simulink model "PFC_MultiAxisKit_Sim"  (R2021b)
settings: Solver=VariableStepAuto  StartTime=0.0  StopTime=0.2  RelTol=1e-3
InitFcn:
  | run('PFC_MultiAxisKit_Param.m')
values from neighbouring files (symbols this model uses):
  f_PWM = 100000    [PFC_MultiAxisKit_Param.m]
  Ts_plant = 2e-7    (= 2e-07)    [PFC_MultiAxisKit_Param.m]
libraries: fl_lib x20, nesl_utility x7, tiiqmathlib x3, c28xdmclib x2, demo_controls x1, ee_lib x1, eePwmGenerator x1
CloseFcn:
  | clear('C_boost','C_filter','f_PWM','fin','L_boost','Ts','Vin_peak','PFC_Results','Ts_control','Ts_plant')
settings Model: Creator=The MathWorks, Inc.  LastModifiedBy=The MathWorks, Inc.
settings SolverCC: AlgebraicLoopSolver=TrustRegion
settings DataIOCC: SaveFormat=StructureWithTime  SaveTime=off  ReturnWorkspaceOutputs=off
settings DebuggingCC: ParameterPrecisionLossMsg=none  SymbolicDimsDataTypeCodeGenerationDiagnostic=none  SFMachineParentedDataDiag=warning

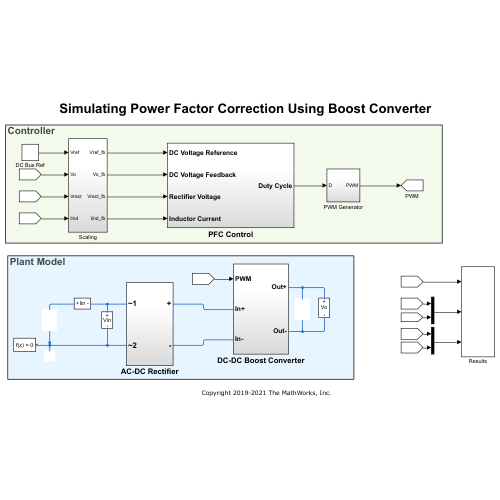
[thumbnail: Simulink's stored preview of the top-level diagram]
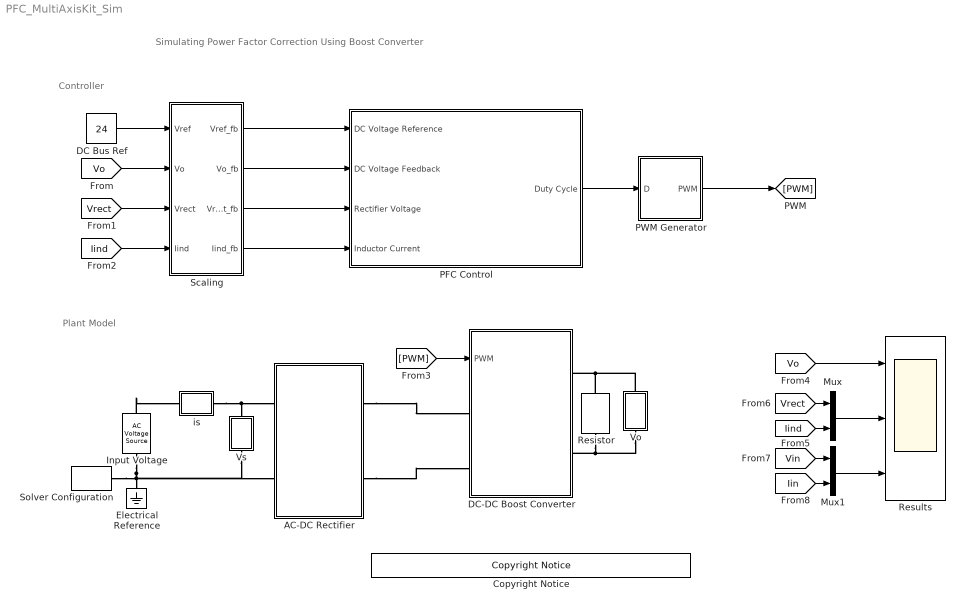
== system PFC_MultiAxisKit_Sim ==
  note: Controller
  note: Plant Model
  note: Simulating Power Factor Correction Using Boost Converter
  AC-DC Rectifier : Subsystem
  Copyright Notice : demo_controls/Copyright Notice  year=2019  prod=tic6000
      settings: SourceProductBaseCode=ME
  DC Bus Ref : Constant  Value=24  SampleTime=2e-5
  DC-DC Boost Converter : Subsystem
  Electrical Reference : fl_lib/Electrical/Electrical Elements/Electrical Reference
  Input Voltage : fl_lib/Electrical/Electrical Sources/AC Voltage Source  amp=Vin_peak V  shift=0 deg  frequency=fin Hz  omega=0 rad/s
  Mux : Mux  Inputs=2
  Mux1 : Mux  Inputs=2
  PFC Control : Subsystem
  PWM Generator : Subsystem
  Resistor : fl_lib/Electrical/Electrical Elements/Resistor  R=15.3 Ohm  i_specify=off  i_priority=None  i=0 A  i_nominal_specify=off  i_nominal_unit=A  i_nominal_value=1  v_specify=off  v_priority=None  v=0 V  v_nominal_specify=off  v_nominal_unit=V  v_nominal_value=1
  Results : Scope  NumInputPorts=3
  Scaling : Subsystem
  Solver Configuration : nesl_utility/Solver Configuration  PhysicalDomain=network_engine_domain  SubClassName=solver  LeftPortType=input  RightPortType=generic  Tones=[]  Harmonics=[]  SimulateNoise=off  Profile=off  UseLocalSampling=off  EnableSwitchedLinearOptims=on  FrequencyDomain=off  UseCCode=off  RelTol=0.001  AbsTol=1e-06  MinStep=1e-09  ToWorkspace=off  RevertToSquareIcSolve=off  NumHomotopyIterations=100  PhasorMode=off  PhasorModeNumHarmonics=1  DoDC=off  ResidualTolerance=1e-09  UseLocalSolver=on  LocalSolverChoice=NE_BACKWARD_EULER_ADVANCER  LocalSolverSampleTime=Ts_plant  DoFixedCost=on  MaxNonlinIter=4  MaxModeIter=2  ComputeImpulses=off  ImpulseIterations=2  LinearAlgebra=auto  EquationFormulation=NE_TIME_EF  DelaysMemoryBudget=1024  AutomaticFiltering=on  FilteringTimeConstant=0.001  PartitionStorageMethod=AS_NEEDED  PartitionMemoryBudget=1024  PartitionMethod=FAST
      settings: SourceProductBaseCode=PW,SS
  Vo : Subsystem
      mask Display:
      | disp('Vo')
      | port_label('Lconn',1,'+')
      | port_label('Rconn',1,'-')
  Vs : Subsystem
      mask Display:
      | disp('Vin')
      | port_label('Lconn',1,'+')
      | port_label('Rconn',1,'-')
  is : Subsystem
      mask Display:
      | disp('Iin')
      | port_label('Lconn',1,'+')
      | port_label('Rconn',1,'-')
  wires:
  PFC Control/1(Duty Cycle) -> PWM Generator/1(D)
  PWM Generator/1(PWM) -> [PWM]
  [Vo] -> Scaling/2(Vo)
  DC Bus Ref/1 -> Scaling/1(Vref)
  [Vrect] -> Scaling/3(Vrect)
  [Iind] -> Scaling/4(Iind)
  [PWM] -> DC-DC Boost Converter/1(PWM)
  Scaling/1(Vref_fb) -> PFC Control/1(DC Voltage Reference)
  [Vo] -> Results/1
  Mux/1 -> Results/2
  Mux1/1 -> Results/3
  [Iind] -> Mux/2
  [Vrect] -> Mux/1
  [Vin] -> Mux1/1
  [Iin] -> Mux1/2
  Scaling/4(Iind_fb) -> PFC Control/4(Inductor Current)
  Scaling/3(Vrect_fb) -> PFC Control/3(Rectifier Voltage)
  Scaling/2(Vo_fb) -> PFC Control/2(DC Voltage Feedback)
  connections:
  Input Voltage/LConn1 -- is/LConn1
  is/RConn1 -- Vs/LConn1 -- AC-DC Rectifier/LConn1
  Input Voltage/RConn1 -- Solver Configuration/RConn1 -- Vs/RConn1 -- AC-DC Rectifier/LConn2 -- Electrical Reference/LConn1
  AC-DC Rectifier/RConn1 -- DC-DC Boost Converter/LConn1
  AC-DC Rectifier/RConn2 -- DC-DC Boost Converter/LConn2
  Resistor/LConn1 -- DC-DC Boost Converter/RConn1 -- Vo/LConn1
  Resistor/RConn1 -- DC-DC Boost Converter/RConn2 -- Vo/RConn1

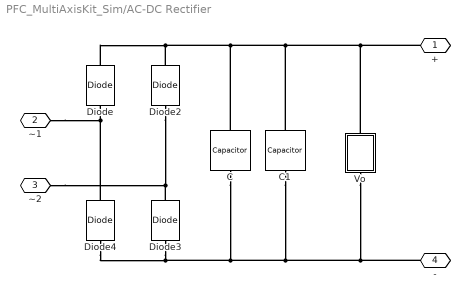
== system PFC_MultiAxisKit_Sim/AC-DC Rectifier ==
  C : fl_lib/Electrical/Electrical Elements/Capacitor  c=220e-9 F  r=1e-6 Ohm  g=0 1/Ohm  i_specify=off  i_priority=None  i=0 A  i_nominal_specify=off  i_nominal_unit=A  i_nominal_value=1  v_specify=off  v_priority=None  v=0 V  v_nominal_specify=off  v_nominal_unit=V  v_nominal_value=1  vc_specify=off  vc_priority=High  vc=0 V  vc_nominal_specify=off  vc_nominal_unit=V  vc_nominal_value=1
  C1 : fl_lib/Electrical/Electrical Elements/Capacitor  c=220e-9 F  r=1e-6 Ohm  g=0 1/Ohm  i_specify=off  i_priority=None  i=0 A  i_nominal_specify=off  i_nominal_unit=A  i_nominal_value=1  v_specify=off  v_priority=None  v=0 V  v_nominal_specify=off  v_nominal_unit=V  v_nominal_value=1  vc_specify=off  vc_priority=High  vc=0 V  vc_nominal_specify=off  vc_nominal_unit=V  vc_nominal_value=1
  Diode{,2..4} (4 alike) : fl_lib/Electrical/Electrical Elements/Diode  Vf=0.8 V  Ron=0.001 Ohm  Goff=1e-8 1/Ohm  i_specify=off  i_priority=None  i=0 A  i_nominal_specify=off  i_nominal_unit=A  i_nominal_value=1  v_specify=off  v_priority=None  v=0 V  v_nominal_specify=off  v_nominal_unit=V  v_nominal_value=1
  Vo : Subsystem
      mask Display:
      | disp('Vrect')
      | port_label('Lconn',1,'+')
      | port_label('Rconn',1,'-')
  + : PMIOPort  Side=Right
  ~1 : PMIOPort  Port=2  Side=Left
  ~2 : PMIOPort  Port=3  Side=Left
  - : PMIOPort  Port=4  Side=Right
  connections:
  Diode3/RConn1 -- ~2/RConn1 -- Diode2/LConn1
  Diode2/RConn1 -- Vo/LConn1 -- +/RConn1 -- C1/LConn1 -- C/LConn1 -- Diode/RConn1
  Diode3/LConn1 -- C/RConn1 -- C1/RConn1 -- Vo/RConn1 -- -/RConn1 -- Diode4/LConn1
  Diode4/RConn1 -- ~1/RConn1 -- Diode/LConn1

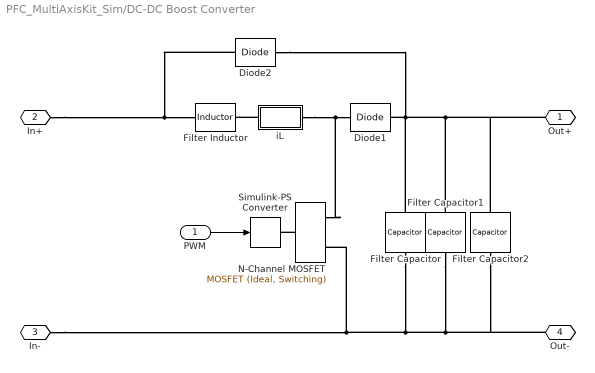
== system PFC_MultiAxisKit_Sim/DC-DC Boost Converter ==
  PWM : Inport
  Diode1 : fl_lib/Electrical/Electrical Elements/Diode  Vf=0.8 V  Ron=0.001 Ohm  Goff=1e-8 1/Ohm  i_specify=off  i_priority=None  i=0 A  i_nominal_specify=off  i_nominal_unit=A  i_nominal_value=1  v_specify=off  v_priority=None  v=0 V  v_nominal_specify=off  v_nominal_unit=V  v_nominal_value=1
  Diode2 : fl_lib/Electrical/Electrical Elements/Diode  Vf=0.8 V  Ron=0.001 Ohm  Goff=1e-8 1/Ohm  i_specify=off  i_priority=None  i=0 A  i_nominal_specify=off  i_nominal_unit=A  i_nominal_value=1  v_specify=off  v_priority=None  v=0 V  v_nominal_specify=off  v_nominal_unit=V  v_nominal_value=1
  Filter Capacitor : fl_lib/Electrical/Electrical Elements/Capacitor  c=47e-9 F  r=1e-6 Ohm  g=0 1/Ohm  i_specify=off  i_priority=None  i=0 A  i_nominal_specify=off  i_nominal_unit=A  i_nominal_value=1  v_specify=off  v_priority=None  v=0 V  v_nominal_specify=off  v_nominal_unit=V  v_nominal_value=1  vc_specify=off  vc_priority=High  vc=0 V  vc_nominal_specify=off  vc_nominal_unit=V  vc_nominal_value=1
  Filter Capacitor1 : fl_lib/Electrical/Electrical Elements/Capacitor  c=C_boost F  r=1e-6 Ohm  g=0 1/Ohm  i_specify=off  i_priority=None  i=0 A  i_nominal_specify=off  i_nominal_unit=A  i_nominal_value=1  v_specify=off  v_priority=None  v=0 V  v_nominal_specify=off  v_nominal_unit=V  v_nominal_value=1  vc_specify=off  vc_priority=High  vc=0 V  vc_nominal_specify=off  vc_nominal_unit=V  vc_nominal_value=1
  Filter Capacitor2 : fl_lib/Electrical/Electrical Elements/Capacitor  c=C_filter F  r=1e-6 Ohm  g=0 1/Ohm  i_specify=off  i_priority=None  i=0 A  i_nominal_specify=off  i_nominal_unit=A  i_nominal_value=1  v_specify=off  v_priority=None  v=0 V  v_nominal_specify=off  v_nominal_unit=V  v_nominal_value=1  vc_specify=off  vc_priority=High  vc=0 V  vc_nominal_specify=off  vc_nominal_unit=V  vc_nominal_value=1
  Filter Inductor : fl_lib/Electrical/Electrical Elements/Inductor  l=L_boost H  r=0.01 Ohm  g=1e-9 1/Ohm  i_specify=off  i_priority=None  i=20 A  i_nominal_specify=off  i_nominal_unit=A  i_nominal_value=1  v_specify=off  v_priority=None  v=0 V  v_nominal_specify=off  v_nominal_unit=V  v_nominal_value=1  i_L_specify=off  i_L_priority=High  i_L=0 A  i_L_nominal_specify=off  i_L_nominal_unit=A  i_L_nominal_value=1
      settings: LogSimulationData=on
  N-Channel MOSFET : ee_lib/Semiconductors & Converters/MOSFET (Ideal, Switching)  Rds=0.22e-6 Ohm  Goff=1e-6 1/Ohm  Vth=0.5 V  diode_param=2  diode_Vf=0.8 V  diode_Ron=0.01 Ohm  diode_Goff=1e-5 1/Ohm  diode_C=5e-8 F  diode_iRM=-235 A  diode_iF=300 A  diode_idot=-50 A/us  diode_trr_param=1  diode_trr_factor=3  diode_trr=15 us  diode_Qrr=1.5e+3 s*uA  thermal_loss_option=ee.enum.converters.thermalLossOption.constantvalues  Von_data=[0, 1.1, 1.3, 1.45, 1.75, 2.25, 2.7; 0, 1, 1.15, 1.35, 1.7, 2.35, 3] V  Tj=[298.15, 398.15] K  Iout_data=[0, 10, 50, 100, 200, 400, 600] A  Eon_data=[0, .29, 1.43, 2.86, 5.71, 13.14, 22.86; 0, .57, 2.63, 5.14, 10.29, 20.57, 30.29] * 1e-3 J  Eoff_data=[0, .21, 1.07, 2.14, 4.29, 9.86, 17.14; 0, .43, 1.97, 3.86, 7.71, 15.43, 22.71] * 1e-3 J  Tj_loss=[298.15, 398.15] K  Iout_data_loss=[0, 10, 50, 100, 200, 400, 600] A  Eon_scalar=22.86e-3 J  Eoff_scalar=17.14e-3 J  Voff=300 V  Iout_scalar=600 A  diodeModelType=ee.enum.converters.diodeModelType.pwl  diodeTableType=ee.enum.diode.tableType.IfMat  diode_IfMat=[.07, .12, .19, 1.75, 4.24, 7.32, 11.2; .16, .3, .72, 2.14, 4.02, 6.35, 9.12] A  diode_VfMat=[.9, 1.15, 1.25, 1.5, 1.75, 2.17, 2.6, 2.85; .58, .68, .75, 1.1, 1.38, 1.77, 2.27, 2.7] V  diode_TjVec=[25, 125] degC  diode_VfVec=[.5, .7, .9, 1.3, 1.7, 2.1, 2.5] V  diode_IfVec=[.1, .2, .5, 1, 2, 4, 7, 10] A  diode_Vr=-600 V  diode_Ls=150 nH  diode_Erec=0.03 J  thermal_network_parameterization=ee.enum.thermalNetworkTopology.external  Rth=[.03, .2] K/W  Rth_Cauer=[.03, .1, .2] K/W  Rth_Foster=[.03, .2] K/W  thermal_mass_parameterization=ee.enum.thermalNetwork.timeconstant  thermal_mass=[3, 25] J/K  thermal_mass_Cauer=[3, 10, 25] J/K  thermal_mass_Foster=[33, 50] J/K  thermal_time_constant=[.1, 5] s  thermal_time_constant_Cauer=[.1, 1, 5] s  thermal_time_constant_Foster=[1, 10] s  thermal_mass_initial_temperatures=[25, 25] degC  thermal_mass_initial_temperatures_Cauer=[25, 25, 25] degC  junction_thermal_mass=0.1 J/K  steadyState_Foster=simscape.enum.onoff.on  Tvec_initial_Foster=[25, 25, 25, 25] degC  no_thermal_network=0  junction_temperature_specify=off  junction_temperature_priority=None  junction_temperature=25 degC  junction_temperature_nominal_specify=off  junction_temperature_nominal_unit=degC  junction_temperature_nominal_value=1  vT_specify=off  vT_priority=None  vT=0 V  vT_nominal_specify=off  vT_nominal_unit=V  vT_nominal_value=1  Qj_specify=off  Qj_priority=None  Qj=0 W  Qj_nominal_specify=off  Qj_nominal_unit=W  Qj_nominal_value=1
  Simulink-PS Converter : nesl_utility/Simulink-PS Converter  PhysicalDomain=network_engine_domain  SubClassName=ps_input  LeftPortType=input  RightPortType=output  PseudoPeriodic=off  Frequencies=[]  NoiseDistribution=none  NoiseParameters=[]  Unit=1  AffineConversion=off  FilteringAndDerivatives=provide  SimscapeFilterOrder=1  InputFilterTimeConstant=0.001  UdotUserProvided=0
      settings: SourceProductBaseCode=PW,SS
  iL : Subsystem
      mask Display:
      | disp('Iind')
      | port_label('Lconn',1,'+')
      | port_label('Rconn',1,'-')
  Out+ : PMIOPort  Side=Right
  In+ : PMIOPort  Port=2  Side=Left
  In- : PMIOPort  Port=3  Side=Left
  Out- : PMIOPort  Port=4  Side=Right
  wires:
  PWM/1 -> Simulink-PS Converter/1
  connections:
  Diode1/RConn1 -- Filter Capacitor2/LConn1 -- Out+/RConn1 -- Filter Capacitor1/LConn1 -- Diode2/RConn1 -- Filter Capacitor/LConn1
  Filter Capacitor/RConn1 -- Filter Capacitor2/RConn1 -- Out-/RConn1 -- Filter Capacitor1/RConn1 -- N-Channel MOSFET/RConn2 -- In-/RConn1
  Diode1/LConn1 -- N-Channel MOSFET/RConn1 -- iL/RConn1
  N-Channel MOSFET/LConn1 -- Simulink-PS Converter/RConn1
  iL/LConn1 -- Filter Inductor/RConn1
  In+/RConn1 -- Diode2/LConn1 -- Filter Inductor/LConn1

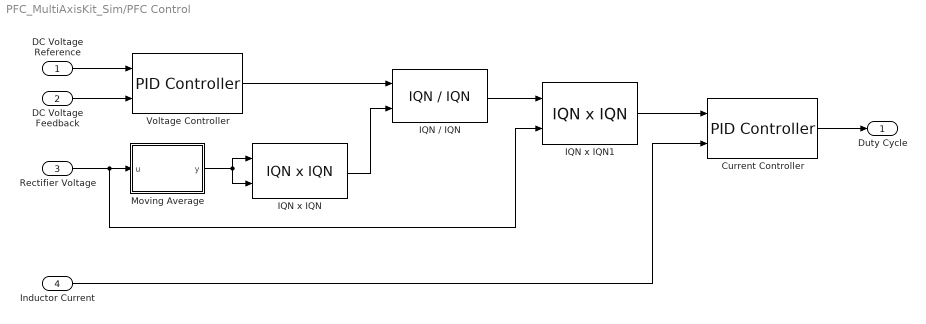
== system PFC_MultiAxisKit_Sim/PFC Control ==
  DC Voltage Reference : Inport
  DC Voltage Feedback : Inport  Port=2
  Rectifier Voltage : Inport  Port=3
  Inductor Current : Inport  Port=4
  Current Controller : c28xdmclib/PID Controller  proportionalGain=0.2776  integralGain=0.10053314  correctionGain=0.3621511  derivativeGain=0  minOutput=0  maxOutput=0.95
      settings: SourceProductBaseCode=TIC2000
  IQN / IQN : tiiqmathlib/IQN // IQN
      settings: SourceProductBaseCode=TIC2000
  IQN x IQN : tiiqmathlib/IQN x IQN  multiplyOption=Multiply
      settings: SourceProductBaseCode=TIC2000
  IQN x IQN1 : tiiqmathlib/IQN x IQN  multiplyOption=Multiply
      settings: SourceProductBaseCode=TIC2000
  Moving Average : MATLAB Function  TreatAsAtomicUnit=on
  Voltage Controller : c28xdmclib/PID Controller  proportionalGain=0.6391  integralGain=0.002513274  correctionGain=0.0039306  derivativeGain=0  minOutput=0  maxOutput=5.11
      settings: SourceProductBaseCode=TIC2000
  Duty Cycle : Outport  VectorParamsAs1DForOutWhenUnconnected=off
  wires:
  Moving Average/1(y) -> IQN x IQN/2, IQN x IQN/1
  Rectifier Voltage/1 -> Moving Average/1(u), IQN x IQN1/2
  IQN / IQN/1 -> IQN x IQN1/1
  IQN x IQN/1 -> IQN / IQN/2
  Inductor Current/1 -> Current Controller/2
  DC Voltage Reference/1 -> Voltage Controller/1
  Voltage Controller/1 -> IQN / IQN/1
  IQN x IQN1/1 -> Current Controller/1
  Current Controller/1 -> Duty Cycle/1
  DC Voltage Feedback/1 -> Voltage Controller/2

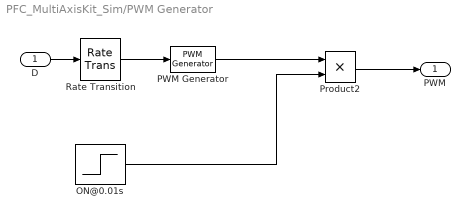
== system PFC_MultiAxisKit_Sim/PWM Generator ==
  D : Inport
  ON@0.01s : Step  Time=0.01  SampleTime=Ts_plant
  PWM Generator : eePwmGenerator/PWM Generator  CarrCount=Up  Tper=1/f_PWM  Tdelay=0  Ts=Ts_plant
  Product2 : Product
  Rate Transition : RateTransition  Deterministic=off
  PWM : Outport  VectorParamsAs1DForOutWhenUnconnected=off
  wires:
  ON@0.01s/1 -> Product2/2
  PWM Generator/1 -> Product2/1
  Product2/1 -> PWM/1
  D/1 -> Rate Transition/1
  Rate Transition/1 -> PWM Generator/1

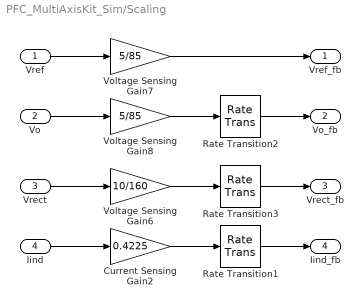
== system PFC_MultiAxisKit_Sim/Scaling ==
  Vref : Inport
  Vo : Inport  Port=2
  Vrect : Inport  Port=3
  Iind : Inport  Port=4
  Current Sensing Gain2 : Gain  Gain=0.4225  OutDataTypeStr=fixdt(1,32,22)
  Rate Transition1 : RateTransition  Integrity=off  Deterministic=off  OutPortSampleTime=Ts_control
  Rate Transition2 : RateTransition  Integrity=off  Deterministic=off  OutPortSampleTime=Ts_control
  Rate Transition3 : RateTransition  Integrity=off  Deterministic=off  OutPortSampleTime=Ts_control
  Voltage Sensing Gain6 : Gain  Gain=10/160  OutDataTypeStr=fixdt(1,32,22)
  Voltage Sensing Gain7 : Gain  Gain=5/85  OutDataTypeStr=fixdt(1,32,22)
  Voltage Sensing Gain8 : Gain  Gain=5/85  OutDataTypeStr=fixdt(1,32,22)
  Vref_fb : Outport  VectorParamsAs1DForOutWhenUnconnected=off
  Vo_fb : Outport  Port=2  VectorParamsAs1DForOutWhenUnconnected=off
  Vrect_fb : Outport  Port=3  VectorParamsAs1DForOutWhenUnconnected=off
  Iind_fb : Outport  Port=4  VectorParamsAs1DForOutWhenUnconnected=off
  wires:
  Iind/1 -> Current Sensing Gain2/1
  Vref/1 -> Voltage Sensing Gain7/1
  Vo/1 -> Voltage Sensing Gain8/1
  Vrect/1 -> Voltage Sensing Gain6/1
  Voltage Sensing Gain7/1 -> Vref_fb/1
  Current Sensing Gain2/1 -> Rate Transition1/1
  Voltage Sensing Gain8/1 -> Rate Transition2/1
  Voltage Sensing Gain6/1 -> Rate Transition3/1
  Rate Transition1/1 -> Iind_fb/1
  Rate Transition2/1 -> Vo_fb/1
  Rate Transition3/1 -> Vrect_fb/1

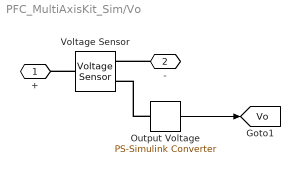
== system PFC_MultiAxisKit_Sim/Vo ==
  Output Voltage : nesl_utility/PS-Simulink Converter  PhysicalDomain=network_engine_domain  SubClassName=ps_output  LeftPortType=input  RightPortType=output  PseudoPeriodic=off  Frequencies=[]  Unit=1  AffineConversion=off
      settings: SourceProductBaseCode=PW,SS
  Voltage Sensor : fl_lib/Electrical/Electrical Sensors/Voltage Sensor
      settings: LogSimulationData=on
  + : PMIOPort  Side=Left
  - : PMIOPort  Port=2  Side=Right
  tag scope: Vo=global
  wires:
  Output Voltage/1 -> [Vo]
  connections:
  Output Voltage/LConn1 -- Voltage Sensor/RConn1
  Voltage Sensor/LConn1 -- +/RConn1
  -/RConn1 -- Voltage Sensor/RConn2

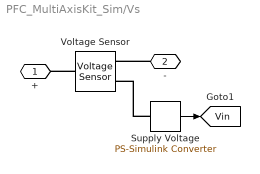
== system PFC_MultiAxisKit_Sim/Vs ==
  Supply Voltage : nesl_utility/PS-Simulink Converter  PhysicalDomain=network_engine_domain  SubClassName=ps_output  LeftPortType=input  RightPortType=output  PseudoPeriodic=off  Frequencies=[]  Unit=1  AffineConversion=off
      settings: SourceProductBaseCode=PW,SS
  Voltage Sensor : fl_lib/Electrical/Electrical Sensors/Voltage Sensor
      settings: LogSimulationData=on
  + : PMIOPort  Side=Left
  - : PMIOPort  Port=2  Side=Right
  tag scope: Vin=global
  wires:
  Supply Voltage/1 -> [Vin]
  connections:
  -/RConn1 -- Voltage Sensor/RConn2
  Voltage Sensor/LConn1 -- +/RConn1
  Supply Voltage/LConn1 -- Voltage Sensor/RConn1

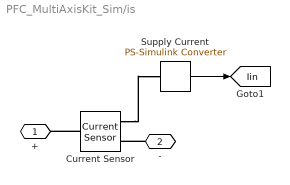
== system PFC_MultiAxisKit_Sim/is ==
  Current Sensor : fl_lib/Electrical/Electrical Sensors/Current Sensor
      settings: LogSimulationData=on
  Supply Current : nesl_utility/PS-Simulink Converter  PhysicalDomain=network_engine_domain  SubClassName=ps_output  LeftPortType=input  RightPortType=output  PseudoPeriodic=off  Frequencies=[]  Unit=1  AffineConversion=off
      settings: SourceProductBaseCode=PW,SS
  + : PMIOPort  Side=Left
  - : PMIOPort  Port=2  Side=Right
  tag scope: Iin=global
  wires:
  Supply Current/1 -> [Iin]
  connections:
  -/RConn1 -- Current Sensor/RConn2
  Current Sensor/RConn1 -- Supply Current/LConn1
  Current Sensor/LConn1 -- +/RConn1

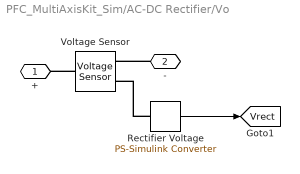
== system PFC_MultiAxisKit_Sim/AC-DC Rectifier/Vo ==
  Rectifier Voltage : nesl_utility/PS-Simulink Converter  PhysicalDomain=network_engine_domain  SubClassName=ps_output  LeftPortType=input  RightPortType=output  PseudoPeriodic=off  Frequencies=[]  Unit=1  AffineConversion=off
      settings: SourceProductBaseCode=PW,SS
  Voltage Sensor : fl_lib/Electrical/Electrical Sensors/Voltage Sensor
      settings: LogSimulationData=on
  + : PMIOPort  Side=Left
  - : PMIOPort  Port=2  Side=Right
  tag scope: Vrect=global
  wires:
  Rectifier Voltage/1 -> [Vrect]
  connections:
  Rectifier Voltage/LConn1 -- Voltage Sensor/RConn1
  Voltage Sensor/LConn1 -- +/RConn1
  -/RConn1 -- Voltage Sensor/RConn2

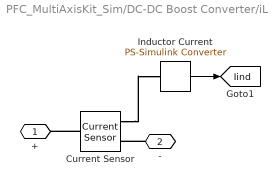
== system PFC_MultiAxisKit_Sim/DC-DC Boost Converter/iL ==
  Current Sensor : fl_lib/Electrical/Electrical Sensors/Current Sensor
  Inductor Current : nesl_utility/PS-Simulink Converter  PhysicalDomain=network_engine_domain  SubClassName=ps_output  LeftPortType=input  RightPortType=output  PseudoPeriodic=off  Frequencies=[]  Unit=1  AffineConversion=off
      settings: SourceProductBaseCode=PW,SS
  + : PMIOPort  Side=Left
  - : PMIOPort  Port=2  Side=Right
  tag scope: Iind=global
  wires:
  Inductor Current/1 -> [Iind]
  connections:
  Current Sensor/LConn1 -- +/RConn1
  Current Sensor/RConn1 -- Inductor Current/LConn1
  -/RConn1 -- Current Sensor/RConn2

== matlab function PFC_MultiAxisKit_Sim/PFC Control/Moving Average ==
  data: u input; y output
function y = fcn(u)

persistent counter;
persistent sum;
persistent out;

if isempty(counter)
    counter = fi(0,1,32,0);
end

if isempty(sum)
    sum = fi(0,1,32,22);
end

if isempty(out)
    out = fi(1,1,32,22);
end

counter = fi(counter + 1,1,32,0);
sum = fi(sum + u,1,32,22);

if (counter == fi(500,1,32,0))
    y = fi(sum/counter,1,32,22);
    out = y;
    sum = fi(0,1,32,22);
    counter = fi(0,1,32,0);
else
    y = out;
end
end
